simulink model "GFLIB_AtanYXShifted_BAM"  (Simulink 9.3)
settings: Solver=VariableStepAuto  StartTime=0.0  StopTime=10.0  RelTol=1e-3
settings Model: Creator=nxa18952  LastModifiedBy=nxa18952
settings DataIOCC: SaveFormat=Dataset  SignalLoggingSaveFormat=Dataset  ReturnWorkspaceOutputs=on
settings OptimizationCC: LifeSpan=auto
settings DebuggingCC: UnderspecifiedInitializationDetection=Simplified  MergeDetectMultiDrivingBlocksExec=error  FcnCallInpInsideContextMsg=error  SFUnexpectedBacktrackingDiag=error  SFNoUnconditionalDefaultTransitionDiag=error  SFExecutionAtInitializationDiag=warning  ArithmeticOperatorsInVariantConditions=error
settings HardwareCC: ProdBitPerPointer=64  ProdBitPerSizeT=64  ProdBitPerPtrDiffT=64  ProdLargestAtomicFloat=Float  ProdIntDivRoundTo=Zero  ProdEndianess=LittleEndian  ProdWordSize=64  ProdHWDeviceType=Intel->x86-64 (Windows64)
settings ModelReferenceCC: PropagateSignalLabelsOutOfModel=on
settings SFSimCC: SimUseLocalCustomCode=on
settings RTWCC: RTWUseLocalCustomCode=on
settings CodeAppCC: StateflowObjectComments=off
settings GRTTargetCC: TargetLangStandard=C99 (ISO)  CombineOutputUpdateFcns=on  GRTInterface=off
settings ConfigComp: CovMetricSettings=dwe  CovHtmlReporting=off  CovSaveCumulativeToWorkspaceVar=off  CovSaveSingleToWorkspaceVar=off  CovExternalEMLEnable=on

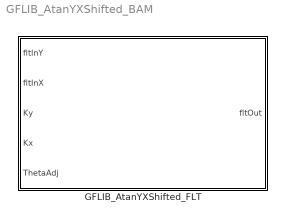
== system GFLIB_AtanYXShifted_BAM ==
  GFLIB_AtanYXShifted_FLT : Subsystem  TreatAsAtomicUnit=on  mask(GFLIB_AtanYXShifted_FLT){}
      mask help: Shifted arctangent of two arguments Y/X in single precision floating-point implementation. Refer to the AMMCLIB User's Guide for further details.
      mask init:
      | if ~evalin('base','exist(''tS8'',''var'')')
      |   if (2 ~= exist('SWLIBS_Typedefs.mat','file'))
      |       error('File SWLIBS_Typedefs.mat is not on the Matlab path. Please add the AMMCLIB "bam" folder in the Matlab Search Path.');
      |   else
      |       evalin('base', 'load(''SWLIBS_Typedefs.mat'')');
      |   end
      | end
      settings: RTWSystemCode=Inline
      mask Display: pos = get_param(gcb, 'Position');width = pos(3) - pos(1); height = pos(4) - pos(2);tX=width/2;tY=height - 8;color('black');text(tX,tY, 'GFLIB_AtanYXShifted_FLT', 'horizontalAlignment', 'center');

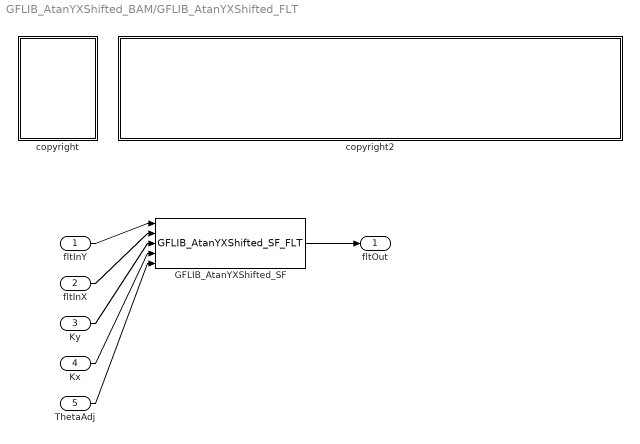
== system GFLIB_AtanYXShifted_BAM/GFLIB_AtanYXShifted_FLT ==
  fltInY : Inport  OutDataTypeStr=single
  fltInX : Inport  Port=2  OutDataTypeStr=single
  Ky : Inport  Port=3  OutDataTypeStr=single
  Kx : Inport  Port=4  OutDataTypeStr=single
  ThetaAdj : Inport  Port=5  OutDataTypeStr=single
  GFLIB_AtanYXShifted_SF : S-Function  FunctionName=GFLIB_AtanYXShifted_SF_FLT  SFunctionDeploymentMode=off  EnableBusSupport=off
  copyright : Subsystem
      mask Display: text(10,90,'FILE:');text(10,75,'DESRIPTION:');text(10,60,'COPYRIGHT:');text(10,45,'VERSION:');text(10,30,'DATE:')
  copyright2 : Subsystem
      mask Display: text(10,90,'GFLIB_AtanYXShifted_BAM_FLT.mdl');text(10,75,'Shifted arctangent of two arguments Y/X.');text(10,60,'NXP 2020');text(10,45,'1.0');text(10,30,'18-Mar-2020');
  fltOut : Outport
  wires:
  fltInY/1 -> GFLIB_AtanYXShifted_SF/1
  fltInX/1 -> GFLIB_AtanYXShifted_SF/2
  Ky/1 -> GFLIB_AtanYXShifted_SF/3
  Kx/1 -> GFLIB_AtanYXShifted_SF/4
  ThetaAdj/1 -> GFLIB_AtanYXShifted_SF/5
  GFLIB_AtanYXShifted_SF/1 -> fltOut/1

== system GFLIB_AtanYXShifted_BAM/GFLIB_AtanYXShifted_FLT/copyright ==

== system GFLIB_AtanYXShifted_BAM/GFLIB_AtanYXShifted_FLT/copyright2 ==
